simulink model "mainDis"  (R2017b)
settings: Solver=VariableStepAuto  StartTime=0.0  StopTime=0.5  FixedStep=2e-4  RelTol=1e-3
values from neighbouring files (symbols this model uses):
  forwardOrder = numel(zero(delta))  - numel(pole(delta))    [calculateDelta.m]    (also in initSim.m = forwardOrderD + forwardOrderF; modelBasedFeedforward.m = numel(zero(feedforwardController)) - numel(pole(feedforwardC)
  Ts = 0.0002    [closedLoopIdentification.m]    (also in initSim.m; test.m)
undefined symbols (not defined in the file or in its folder): forwardOrderD
libraries: cstblocks x4, model_controller x3
settings Model: Creator=Dai Luyao  LastModifiedBy=Princess
settings CodeAppCC: StateflowObjectComments=on

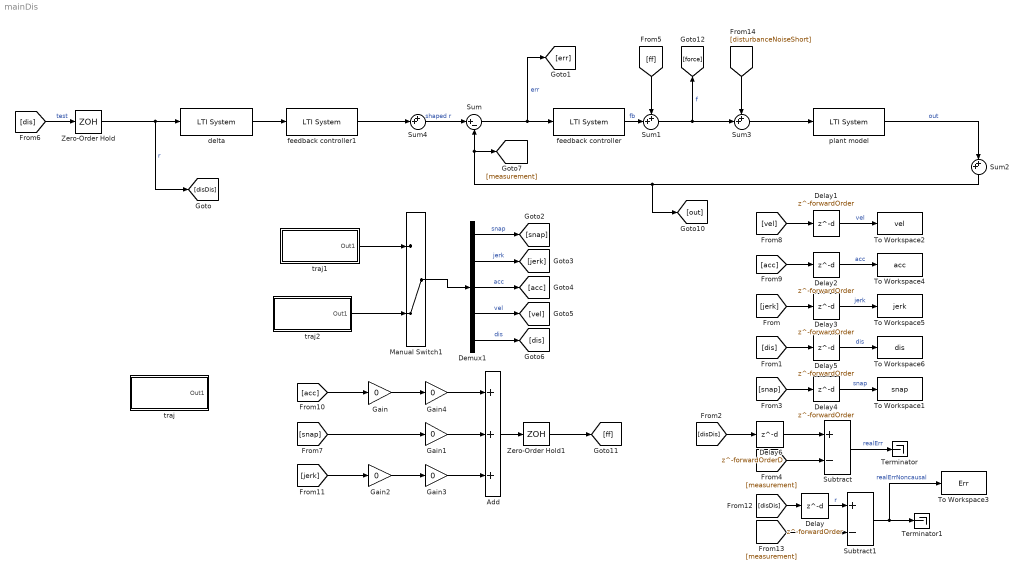
== system mainDis ==
  Add : Sum  Inputs=+++
  Delay{,1..5} (6 alike) : Delay  DelayLength=forwardOrder  SampleTime=Ts
  Delay6 : Delay  DelayLength=forwardOrderD  SampleTime=Ts
  Demux1 : Demux  Outputs=5
  Gain{,1..4} (5 alike) : Gain  Gain=0
  Manual Switch1 : ManualSwitch  CurrentSetting=0
  Subtract : Sum  Inputs=+-
  Subtract1 : Sum  Inputs=+-
  Sum : Sum  Inputs=|+-
  Sum{1..4} (4 alike) : Sum  Inputs=++|
  Terminator : Terminator
  Terminator1 : Terminator
  To Workspace1 : ToWorkspace  VariableName=snap  SaveFormat=Structure With Time  SampleTime=-1
  To Workspace2 : ToWorkspace  VariableName=vel  SaveFormat=Structure With Time  SampleTime=-1
  To Workspace3 : ToWorkspace  VariableName=Err  SaveFormat=Structure With Time  SampleTime=-1
  To Workspace4 : ToWorkspace  VariableName=acc  SaveFormat=Structure With Time  SampleTime=-1
  To Workspace5 : ToWorkspace  VariableName=jerk  SaveFormat=Structure With Time  SampleTime=-1
  To Workspace6 : ToWorkspace  VariableName=dis  SaveFormat=Structure With Time  SampleTime=-1
  Zero-Order Hold : ZeroOrderHold  SampleTime=Ts
  Zero-Order Hold1 : ZeroOrderHold  SampleTime=Ts
  delta : cstblocks/LTI System  sys=deltaCausal  IC=[]
  feedback controller : cstblocks/LTI System  sys=GcDis  IC=[]
  feedback controller1 : cstblocks/LTI System  sys=FCausal  IC=[]
  plant model : cstblocks/LTI System  sys=GpDis  IC=[]
  traj : Subsystem  BlockChoice=4th order traj
      link override 2nd order traj: Ts=Ts
      link override 3rd order traj: j=800  v=0.25  x=0.06  a=10
      link override 4th order traj: a=10  v=0.25  x=0.04  j=800  d=64000  Ts=Ts
      settings: AttributesFormatString=%<BlockChoice>  TemplateBlock=model_controller/Profile Generators/traj  MemberBlocks=2th order traj,3rd order traj,4th order traj,step
  traj1 : Subsystem  BlockChoice=4th order traj
      link override 3rd order traj: j=800  v=0.25  x=0.06  a=10
      link override 4th order traj: a=20  v=0.5  x=0.2  j=2000  d=1.5e6
      settings: AttributesFormatString=%<BlockChoice>  TemplateBlock=model_controller/Profile Generators/traj  MemberBlocks=2th order traj,3rd order traj,4th order traj,step
  traj2 : Subsystem  BlockChoice=4th order traj
      link override 2nd order traj: Ts=Ts
      link override 3rd order traj: j=800  v=0.25  x=0.06  a=10
      link override 4th order traj: a=30  v=0.6  x=0.04  j=2000  d=1000000  Ts=Ts
      settings: AttributesFormatString=%<BlockChoice>  TemplateBlock=model_controller/Profile Generators/traj  MemberBlocks=2th order traj,3rd order traj,4th order traj,step
  wires:
  Sum/1 -> feedback controller/1, [err]  "err"
  feedback controller/1 -> Sum1/2  "fb"
  Sum1/1 -> Sum3/2, [force]  "f"
  plant model/1 -> Sum2/2  "out"
  Demux1/1 -> [snap]  "snap"
  Demux1/2 -> [jerk]  "jerk"
  Demux1/3 -> [acc]  "acc"
  Demux1/4 -> [vel]  "vel"
  Demux1/5 -> [dis]  "dis"
  [acc] -> Gain/1
  Zero-Order Hold/1 -> [disDis], delta/1  "r"
  [ff] -> Sum1/1
  [snap] -> Gain1/1
  Gain/1 -> Gain4/1
  Gain1/1 -> Add/2
  traj1/1(Out1) -> Manual Switch1/1
  Manual Switch1/1 -> Demux1/1
  Add/1 -> Zero-Order Hold1/1
  Zero-Order Hold1/1 -> [ff]
  Sum2/1 -> [out], Sum/2, [measurement]
  Gain2/1 -> Gain3/1
  [jerk] -> Gain2/1
  Gain3/1 -> Add/3
  Gain4/1 -> Add/1
  Sum3/1 -> plant model/1
  [measurement] -> Subtract/2
  Subtract/1 -> Terminator/1  "realErr"
  Subtract1/1 -> To Workspace3/1, Terminator1/1  "realErrNoncausal"
  [measurement] -> Subtract1/2
  [disDis] -> Delay/1
  Delay/1 -> Subtract1/1  "r"
  [disturbanceNoiseShort] -> Sum3/1
  [dis] -> Zero-Order Hold/1  "test"
  feedback controller1/1 -> Sum4/2
  Sum4/1 -> Sum/1  "shaped r"
  delta/1 -> feedback controller1/1
  [vel] -> Delay1/1
  Delay1/1 -> To Workspace2/1  "vel"
  [acc] -> Delay2/1
  Delay2/1 -> To Workspace4/1  "acc"
  [jerk] -> Delay3/1
  Delay3/1 -> To Workspace5/1  "jerk"
  [snap] -> Delay4/1
  Delay4/1 -> To Workspace1/1  "snap"
  [dis] -> Delay5/1
  Delay5/1 -> To Workspace6/1  "dis"
  traj2/1(Out1) -> Manual Switch1/2
  [disDis] -> Delay6/1
  Delay6/1 -> Subtract/1

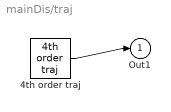
== system mainDis/traj ==
  4th order traj : model_controller/Profile Generators/4th order traj  t0=0  x=0.04  v=0.25  a=10  j=800  d=64000  Ts=Ts
  Out1 : Outport
  wires:
  4th order traj/1 -> Out1/1

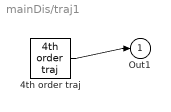
== system mainDis/traj1 ==
  4th order traj : model_controller/Profile Generators/4th order traj  t0=0  x=0.2  v=0.5  a=20  j=2000  d=1.5e6  Ts=0
  Out1 : Outport
  wires:
  4th order traj/1 -> Out1/1

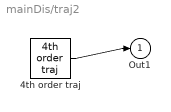
== system mainDis/traj2 ==
  4th order traj : model_controller/Profile Generators/4th order traj  t0=0  x=0.04  v=0.6  a=30  j=2000  d=1000000  Ts=Ts
  Out1 : Outport
  wires:
  4th order traj/1 -> Out1/1
